simulink model "sim_lead_vs_leadlag2"  (R2023b)
settings: Solver=ode8  StartTime=0.0  StopTime=15  FixedStep=0.001  RelTol=1e-3
values from neighbouring files (symbols this model uses):
  K = p/z    [lead_vs_leadlag.m]    (also in setup_lead_controller.m)
  p = bodeoptions    [PID_lead_linmod.m]    (also in lead_vs_leadlag.m = 1/(alpha*T); setup_lead_controller.m = 1/(alpha*T))
  p2 = 0.01    [lead_vs_leadlag.m]
  z = 1/T    [lead_vs_leadlag.m]    (also in setup_lead_controller.m)
  z2 = 0.1    [lead_vs_leadlag.m]
libraries: simulink x1
settings Model: Creator=suvo  LastModifiedBy=suvo
settings SolverCC: AlgebraicLoopSolver=TrustRegion
settings DataIOCC: ReturnWorkspaceOutputs=off
settings DebuggingCC: UnconnectedInputMsg=warning  UnconnectedOutputMsg=warning  UnconnectedLineMsg=warning
settings ModelReferenceCC: EnableRefExpFcnMdlSchedulingChecks=on

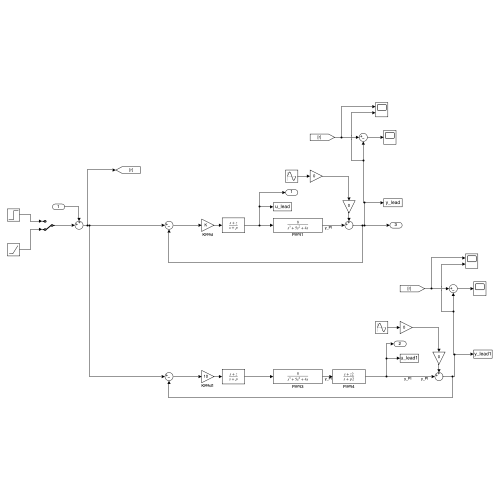
[thumbnail: Simulink's stored preview of the top-level diagram]
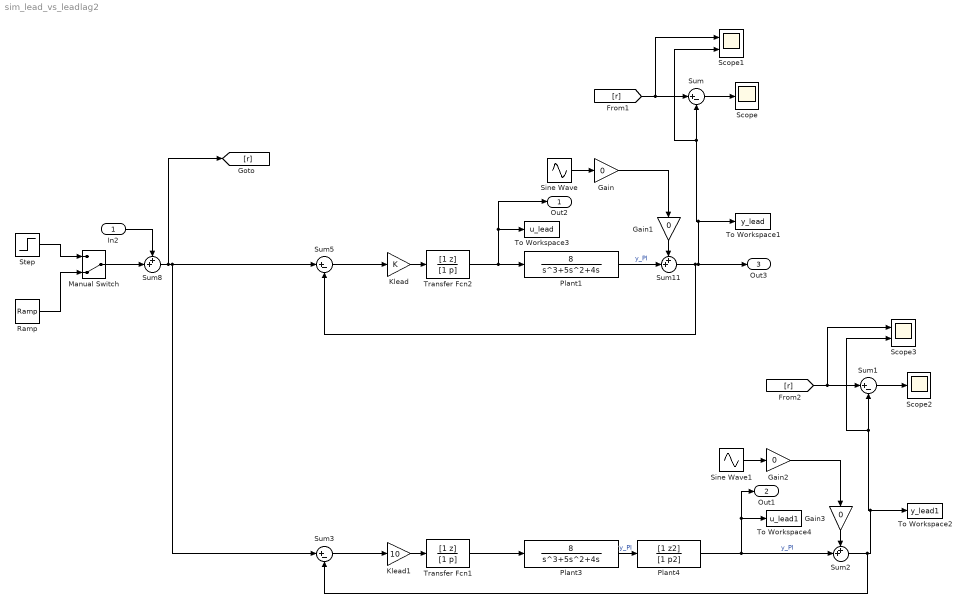
== system sim_lead_vs_leadlag2 ==
  In2 : Inport
  Gain{,1..3} (4 alike) : Gain  Gain=0
  Klead : Gain  Gain=K
  Klead1 : Gain  Gain=10
  Manual Switch : ManualSwitch  CurrentSetting=0
  Plant1 : TransferFcn  Numerator=8  Denominator=[1 5 4 0]
  Plant3 : TransferFcn  Numerator=8  Denominator=[1 5 4 0]
  Plant4 : TransferFcn  Numerator=[1 z2]  Denominator=[1 p2]
  Ramp : simulink/Sources/Ramp  slope=1  start=0  InitialOutput=0
  Scope : Scope
  Scope1 : Scope  NumInputPorts=2
  Scope2 : Scope
  Scope3 : Scope  NumInputPorts=2
  Sine Wave : Sin  Amplitude=0.001  Frequency=50  SampleTime=0
  Sine Wave1 : Sin  Amplitude=0.001  Frequency=50  SampleTime=0
  Step : Step  SampleTime=0
  Sum{,1,3,5} (4 alike) : Sum  Inputs=|+-
  Sum11 : Sum  Inputs=++|
  Sum2 : Sum  Inputs=++|
  Sum8 : Sum  Inputs=++|
  To Workspace1 : ToWorkspace  VariableName=y_lead  SaveFormat=Timeseries  SampleTime=-1
  To Workspace2 : ToWorkspace  VariableName=y_lead1  SaveFormat=Timeseries  SampleTime=-1
  To Workspace3 : ToWorkspace  VariableName=u_lead  SaveFormat=Timeseries  SampleTime=-1
  To Workspace4 : ToWorkspace  VariableName=u_lead1  SaveFormat=Timeseries  SampleTime=-1
  Transfer Fcn1 : TransferFcn  Numerator=[1 z]  Denominator=[1 p]
  Transfer Fcn2 : TransferFcn  Numerator=[1 z]  Denominator=[1 p]
  Out2 : Outport
  Out1 : Outport  Port=2
  Out3 : Outport  Port=3
  wires:
  In2/1 -> Sum8/1
  Plant1/1 -> Sum11/2  "y_PI"
  Sum11/1 -> Out3/1, To Workspace1/1, Scope1/2, Sum/2, Sum5/2
  Gain/1 -> Gain1/1
  Sine Wave/1 -> Gain/1
  Transfer Fcn2/1 -> Plant1/1, Out2/1, To Workspace3/1
  Klead/1 -> Transfer Fcn2/1
  Gain1/1 -> Sum11/1
  [r] -> Scope1/1, Sum/1
  Sum/1 -> Scope/1
  Sum1/1 -> Scope2/1
  Klead1/1 -> Transfer Fcn1/1
  Gain2/1 -> Gain3/1
  Sine Wave1/1 -> Gain2/1
  [r] -> Scope3/1, Sum1/1
  Sum2/1 -> To Workspace2/1, Scope3/2, Sum1/2, Sum3/2
  Sum3/1 -> Klead1/1
  Gain3/1 -> Sum2/1
  Transfer Fcn1/1 -> Plant3/1
  Manual Switch/1 -> Sum8/2
  Ramp/1 -> Manual Switch/2
  Step/1 -> Manual Switch/1
  Sum5/1 -> Klead/1
  Sum8/1 -> Sum3/1, Sum5/1, [r]
  Plant3/1 -> Plant4/1  "y_PI"
  Plant4/1 -> Sum2/2, Out1/1, To Workspace4/1  "y_PI"
